simulink model "task1_model"  (R2021b)
settings: Solver=FixedStepAuto  StartTime=0.0  StopTime=5  FixedStep=timeStep  RelTol=1e-3
undefined symbols (not defined in the file): A, B, C, x1, x2, x3, x4
libraries: simulink x1
settings Model: Creator=den  LastModifiedBy=den

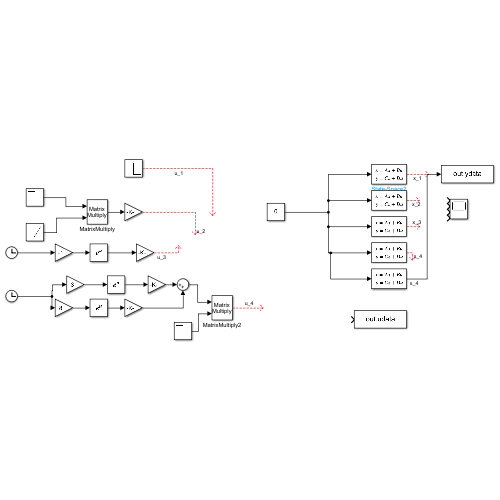
[thumbnail: Simulink's stored preview of the top-level diagram]
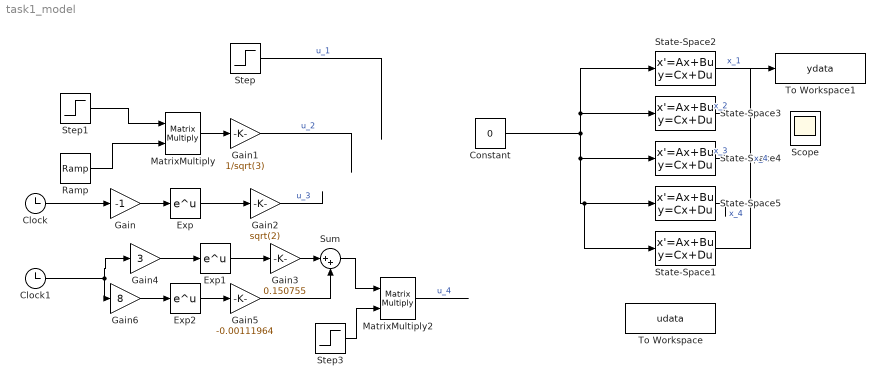
== system task1_model ==
  Clock : Clock
  Clock1 : Clock
  Constant : Constant  Value=0
  Exp : Math  SaturateOnIntegerOverflow=on
  Exp1 : Math  SaturateOnIntegerOverflow=on
  Exp2 : Math  SaturateOnIntegerOverflow=on
  Gain : Gain  Gain=-1
  Gain1 : Gain  Gain=1/sqrt(3)
  Gain2 : Gain  Gain=sqrt(2)
  Gain3 : Gain  Gain=0.150755
  Gain4 : Gain  Gain=3
  Gain5 : Gain  Gain=-0.00111964
  Gain6 : Gain  Gain=8
  MatrixMultiply : Product  Multiplication=Matrix(*)
  MatrixMultiply2 : Product  Multiplication=Matrix(*)
  Ramp : simulink/Sources/Ramp  slope=-1  start=0  InitialOutput=1
  Scope : Scope  NumInputPorts=4
  State-Space1 : StateSpace  A=A  B=B  C=C  D=[0; 0]  InitialCondition=[0.2; 0.1]
  State-Space2 : StateSpace  A=A  B=B  C=C  D=[0; 0]  InitialCondition=x1
  State-Space3 : StateSpace  A=A  B=B  C=C  D=[0; 0]  InitialCondition=x2
  State-Space4 : StateSpace  A=A  B=B  C=C  D=[0; 0]  InitialCondition=x3
  State-Space5 : StateSpace  A=A  B=B  C=C  D=[0; 0]  InitialCondition=x4
  Step : Step  Before=1  After=0  SampleTime=0
  Step1 : Step  Time=3  Before=1  After=0  SampleTime=0
  Step3 : Step  Time=1.1196826  Before=1  After=0  SampleTime=0
  Sum : Sum  Inputs=|++
  To Workspace : ToWorkspace  VariableName=udata  SaveFormat=Structure  SampleTime=-1
  To Workspace1 : ToWorkspace  VariableName=ydata  SaveFormat=Structure  SampleTime=-1
  wires:
  Step/1 -> ?  "u_1"
  Ramp/1 -> MatrixMultiply/2
  MatrixMultiply/1 -> Gain1/1
  Clock/1 -> Gain/1
  Exp/1 -> Gain2/1
  Gain/1 -> Exp/1
  Step1/1 -> MatrixMultiply/1
  Gain1/1 -> ?  "u_2"
  Gain2/1 -> ?  "u_3"
  Gain4/1 -> Exp1/1
  Exp1/1 -> Gain3/1
  Gain3/1 -> Sum/1
  Gain6/1 -> Exp2/1
  Exp2/1 -> Gain5/1
  Gain5/1 -> Sum/2
  Sum/1 -> MatrixMultiply2/1
  Clock1/1 -> Gain4/1, Gain6/1
  Step3/1 -> MatrixMultiply2/2
  MatrixMultiply2/1 -> ?  "u_4"
  State-Space2/1 -> ?  "x_1"
  Constant/1 -> State-Space1/1, State-Space5/1, State-Space4/1, State-Space3/1, State-Space2/1
  State-Space3/1 -> ?  "x_2"
  State-Space4/1 -> ?  "x_3"
  State-Space5/1 -> ?  "x_4"
  State-Space1/1 -> To Workspace1/1  "x_4"
